simulink model "pure_pursuit_sl"  (R2019a)
settings: Solver=FixedStepDiscrete  StartTime=0.0  StopTime=inf  FixedStep=0.01  RelTol=1e-3
model workspace (MAT data in the model file):
  SL_ROS_VariableLengthArrays_MaxSizes.CommonInfo.ArrayTruncateAction = 'EmitWarning'
  SL_ROS_VariableLengthArrays_MaxSizes.MsgTypeMap = containers.Map
  SL_ROS_VariableLengthArrays_MaxSizes.MsgTypeMap.serialization.keys = {'autoware_msgs/Lane', 'autoware_msgs/lane', 'visualization_msgs/Marker'}
  SL_ROS_VariableLengthArrays_MaxSizes.MsgTypeMap.serialization.values{1}.PropertyName = 'Waypoints'
  SL_ROS_VariableLengthArrays_MaxSizes.MsgTypeMap.serialization.values{1}.DataType = 'autoware_msgs/Waypoint'
  SL_ROS_VariableLengthArrays_MaxSizes.MsgTypeMap.serialization.values{1}.MaxLength = 101
  SL_ROS_VariableLengthArrays_MaxSizes.MsgTypeMap.serialization.values{2}.PropertyName = 'Waypoints'
  SL_ROS_VariableLengthArrays_MaxSizes.MsgTypeMap.serialization.values{2}.DataType = 'autoware_msgs/waypoint'
  SL_ROS_VariableLengthArrays_MaxSizes.MsgTypeMap.serialization.values{2}.MaxLength = 101
  SL_ROS_VariableLengthArrays_MaxSizes.MsgTypeMap.serialization.values{3}(1).PropertyName = 'Colors'
  SL_ROS_VariableLengthArrays_MaxSizes.MsgTypeMap.serialization.values{3}(1).DataType = 'std_msgs/ColorRGBA'
  SL_ROS_VariableLengthArrays_MaxSizes.MsgTypeMap.serialization.values{3}(1).MaxLength = 80
  SL_ROS_VariableLengthArrays_MaxSizes.MsgTypeMap.serialization.values{3}(2).PropertyName = 'MeshResource'
  SL_ROS_VariableLengthArrays_MaxSizes.MsgTypeMap.serialization.values{3}(2).DataType = 'uint8'
  SL_ROS_VariableLengthArrays_MaxSizes.MsgTypeMap.serialization.values{3}(2).MaxLength = 128
  SL_ROS_VariableLengthArrays_MaxSizes.MsgTypeMap.serialization.values{3}(3).PropertyName = 'Ns'
  SL_ROS_VariableLengthArrays_MaxSizes.MsgTypeMap.serialization.values{3}(3).DataType = 'uint8'
  SL_ROS_VariableLengthArrays_MaxSizes.MsgTypeMap.serialization.values{3}(3).MaxLength = 128
  SL_ROS_VariableLengthArrays_MaxSizes.MsgTypeMap.serialization.values{3}(4).PropertyName = 'Points'
  SL_ROS_VariableLengthArrays_MaxSizes.MsgTypeMap.serialization.values{3}(4).DataType = 'geometry_msgs/Point'
  SL_ROS_VariableLengthArrays_MaxSizes.MsgTypeMap.serialization.values{3}(4).MaxLength = 80
  SL_ROS_VariableLengthArrays_MaxSizes.MsgTypeMap.serialization.values{3}(5).PropertyName = 'Text'
  SL_ROS_VariableLengthArrays_MaxSizes.MsgTypeMap.serialization.values{3}(5).DataType = 'uint8'
  SL_ROS_VariableLengthArrays_MaxSizes.MsgTypeMap.serialization.values{3}(5).MaxLength = 128
  SL_ROS_VariableLengthArrays_MaxSizes.MsgTypeMap.serialization.uniformity = 0
  SL_ROS_VariableLengthArrays_MaxSizes.MsgTypeMap.serialization.keyType = 'char'
  SL_ROS_VariableLengthArrays_MaxSizes.MsgTypeMap.serialization.valueType = 'any'
  is_pose_set_ = Simulink.Signal
  is_pose_set_.DataType = 'boolean'
  is_pose_set_.Dimensions = 1
  is_pose_set_.DimensionsMode = 'Fixed'
  is_pose_set_.Complexity = 'real'
  is_pose_set_.SampleTime = -1
  is_pose_set_.SamplingMode = 'auto'
  is_pose_set_.InitialValue = 'false'
  is_velocity_set_ = Simulink.Signal
  is_velocity_set_.DataType = 'boolean'
  is_velocity_set_.Dimensions = 1
  is_velocity_set_.DimensionsMode = 'Fixed'
  is_velocity_set_.Complexity = 'real'
  is_velocity_set_.SampleTime = -1
  is_velocity_set_.SamplingMode = 'auto'
  is_velocity_set_.InitialValue = 'false'
  is_waypoint_set_ = Simulink.Signal
  is_waypoint_set_.DataType = 'boolean'
  is_waypoint_set_.Dimensions = 1
  is_waypoint_set_.DimensionsMode = 'Fixed'
  is_waypoint_set_.Complexity = 'real'
  is_waypoint_set_.SampleTime = -1
  is_waypoint_set_.SamplingMode = 'auto'
  is_waypoint_set_.InitialValue = 'false'
  minimum_lookahead_distance = Simulink.Parameter
  minimum_lookahead_distance.Value = 6
  minimum_lookahead_distance.DataType = 'auto'
  minimum_lookahead_distance.Dimensions = [1 1]
undefined symbols (not defined in the file): Action, Color, Colors, Colors_SL_Info, FrameLocked, Header, Id, Ns, Points, Points_SL_Info, Pose, Scale, Twist, Type, X, Y, Z
libraries: robotlib x22, robotcorelib x4, simulink x1
(part 1 of 2)
settings Model: Creator=handai  LastModifiedBy=root
settings DataIOCC: SaveOutput=off  SignalLogging=off  DSMLogging=off  SaveTime=off  ReturnWorkspaceOutputs=off
settings DebuggingCC: PregeneratedLibrarySubsystemCodeDiagnostic=none  ArithmeticOperatorsInVariantConditions=warning
settings SFSimCC: SimUseLocalCustomCode=off
settings RTWCC: RTWUseLocalCustomCode=off

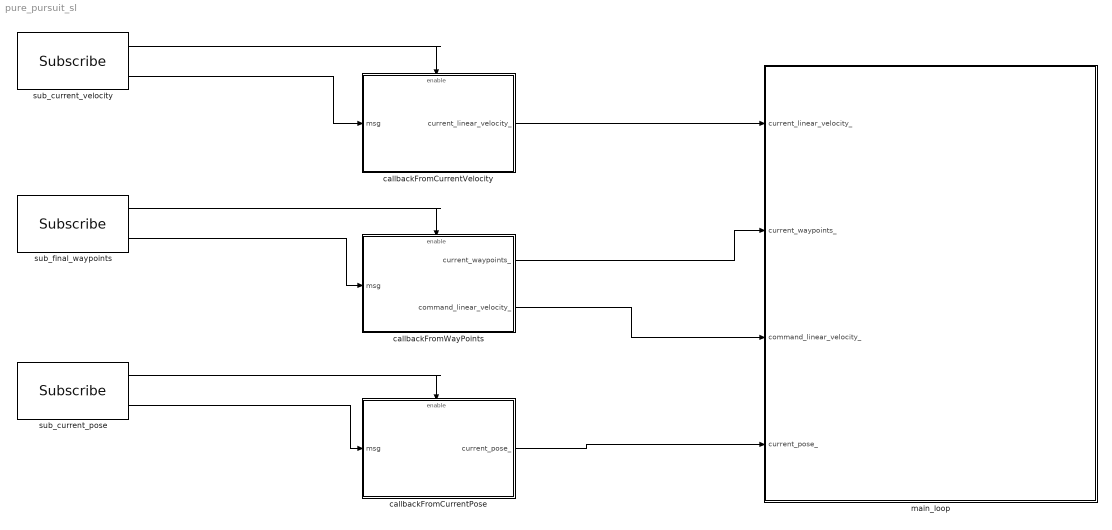
== system pure_pursuit_sl ==
  callbackFromCurrentPose : Subsystem
  callbackFromCurrentVelocity : Subsystem
  callbackFromWayPoints : Subsystem
  main_loop : Subsystem  TreatAsAtomicUnit=on  SystemSampleTime=0.03
      settings: AttributesFormatString=Ts = %<SystemSampleTime>[s]
  sub_current_pose : robotlib/Subscribe  topicSource=Specify your own  topic=/current_pose  messageType=geometry_msgs/PoseStamped  sampleTime=0.01  messageQueueLength=1
      settings: AttributesFormatString=Ts = %<sampleTime>[s]  SourceProductBaseCode=RO
  sub_current_velocity : robotlib/Subscribe  topicSource=Specify your own  topic=/current_velocity  messageType=geometry_msgs/TwistStamped  sampleTime=0.01  messageQueueLength=1
      settings: AttributesFormatString=Ts = %<sampleTime>[s]  SourceProductBaseCode=RO
  sub_final_waypoints : robotlib/Subscribe  topicSource=Specify your own  topic=/final_waypoints  messageType=autoware_msgs/Lane  sampleTime=-1  messageQueueLength=1
      settings: AttributesFormatString=Ts = %<sampleTime>[s]  SourceProductBaseCode=RO
  wires:
  sub_final_waypoints/1 -> callbackFromWayPoints/Enable
  sub_current_pose/2 -> callbackFromCurrentPose/1(msg)
  sub_current_pose/1 -> callbackFromCurrentPose/Enable
  sub_final_waypoints/2 -> callbackFromWayPoints/1(msg)
  callbackFromWayPoints/2(command_linear_velocity_) -> main_loop/3(command_linear_velocity_)
  sub_current_velocity/2 -> callbackFromCurrentVelocity/1(msg)
  sub_current_velocity/1 -> callbackFromCurrentVelocity/Enable
  callbackFromCurrentVelocity/1(current_linear_velocity_) -> main_loop/1(current_linear_velocity_)
  callbackFromWayPoints/1(current_waypoints_) -> main_loop/2(current_waypoints_)
  callbackFromCurrentPose/1(current_pose_) -> main_loop/4(current_pose_)

== system pure_pursuit_sl/callbackFromCurrentPose ==
  msg : Inport
  Enable : EnablePort
  Bus Selector : BusSelector  OutputSignals=Pose
  Constant : Constant  Value=true
  Data Store Write : DataStoreWrite  DataStoreName=is_pose_set_
  Signal Conversion1 : SignalConversion  OverrideOpt=off
  current_pose_ : Outport
  wires:
  Bus Selector/1 -> Signal Conversion1/1  "<Pose>"
  msg/1 -> Bus Selector/1
  Signal Conversion1/1 -> current_pose_/1  "current_pose_"
  Constant/1 -> Data Store Write/1

== system pure_pursuit_sl/callbackFromCurrentVelocity ==
  msg : Inport
  Enable : EnablePort
  Bus Selector1 : BusSelector  OutputSignals=Twist.Linear.X
  Constant : Constant  Value=true
  Data Store Write : DataStoreWrite  DataStoreName=is_velocity_set_
  Signal Conversion : SignalConversion  OverrideOpt=off
  current_linear_velocity_ : Outport
  wires:
  Bus Selector1/1 -> Signal Conversion/1  "<X>"
  msg/1 -> Bus Selector1/1
  Signal Conversion/1 -> current_linear_velocity_/1  "current_linear_velocity_"
  Constant/1 -> Data Store Write/1

== system pure_pursuit_sl/callbackFromWayPoints ==
  msg : Inport
  Enable : EnablePort
  Constant : Constant  Value=true
  Data Store Write : DataStoreWrite  DataStoreName=is_waypoint_set_
  Selector : Selector  IndexMode=Zero-based  InputPortWidth=101  IndexOptions=Index vector (port)  Indices=[1 3]  OutputSizes=1
  Signal Conversion2 : SignalConversion  OverrideOpt=off
  Signal Conversion3 : SignalConversion  OverrideOpt=off
  command_linear_velocity : BusSelector  OutputSignals=Twist.Twist.Linear.X
  idx : Constant  Value=0
  waypoint1 : BusSelector  OutputSignals=Waypoints
  current_waypoints_ : Outport
  command_linear_velocity_ : Outport  Port=2
  wires:
  waypoint1/1 -> Signal Conversion3/1, Selector/1  "<Waypoints>"
  Signal Conversion2/1 -> command_linear_velocity_/1  "command_linear_velocity_"
  idx/1 -> Selector/2
  command_linear_velocity/1 -> Signal Conversion2/1  "<X>"
  msg/1 -> waypoint1/1
  Selector/1 -> command_linear_velocity/1
  Signal Conversion3/1 -> current_waypoints_/1  "current_waypoints_"
  Constant/1 -> Data Store Write/1

== system pure_pursuit_sl/main_loop ==
  current_linear_velocity_ : Inport
  current_waypoints_ : Inport  Port=2
  command_linear_velocity_ : Inport  Port=3
  current_pose_ : Inport  Port=4
  Data Store Read : DataStoreRead  DataStoreName=is_pose_set_
  Data Store Read1 : DataStoreRead  DataStoreName=is_velocity_set_
  Data Store Read2 : DataStoreRead  DataStoreName=is_waypoint_set_
  If1 : If  NumInputs=3  IfExpression=u1 | u2 | u3
  Logical Operator : Logic  Operator=NOT  AllPortsSameDT=off  OutDataTypeStr=boolean
  Logical Operator1 : Logic  Operator=NOT  AllPortsSameDT=off  OutDataTypeStr=boolean
  Logical Operator2 : Logic  Operator=NOT  AllPortsSameDT=off  OutDataTypeStr=boolean
  loop_action : Subsystem  TreatAsAtomicUnit=on
  warn_messge : Subsystem  TreatAsAtomicUnit=on
  wires:
  Data Store Read/1 -> Logical Operator/1
  Data Store Read1/1 -> Logical Operator1/1
  Data Store Read2/1 -> Logical Operator2/1
  Logical Operator2/1 -> If1/3
  Logical Operator1/1 -> If1/2
  Logical Operator/1 -> If1/1
  If1/1 -> warn_messge/Action
  If1/2 -> loop_action/Action
  current_linear_velocity_/1 -> loop_action/1(current_linear_velocity_)
  current_waypoints_/1 -> loop_action/2(current_waypoints_)
  command_linear_velocity_/1 -> loop_action/3(command_linear_velocity_)
  current_pose_/1 -> loop_action/4(current_pose_)

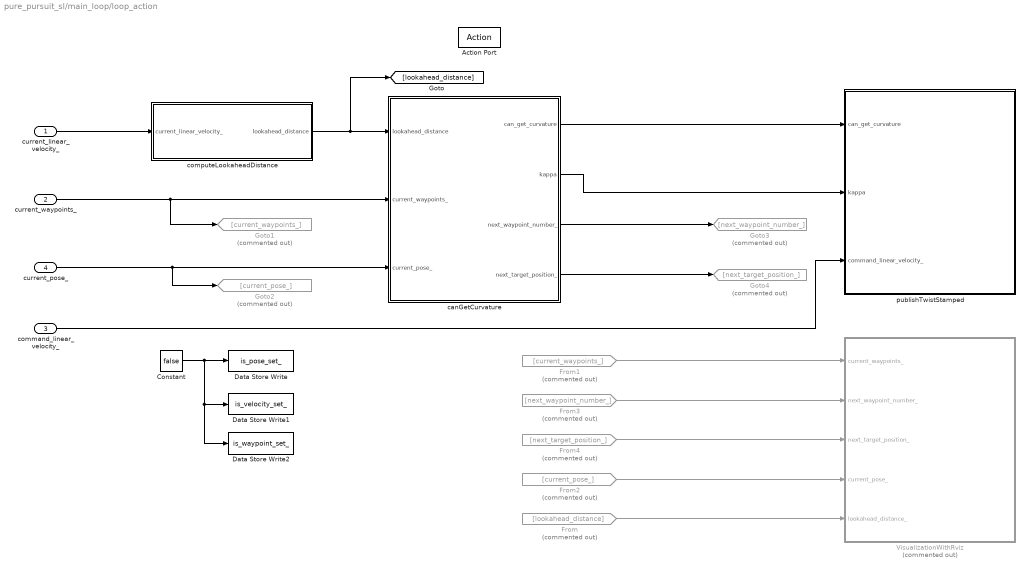
== system pure_pursuit_sl/main_loop/loop_action ==
  current_linear_velocity_ : Inport
  current_waypoints_ : Inport  Port=2
  command_linear_velocity_ : Inport  Port=3
  current_pose_ : Inport  Port=4
  Action Port : ActionPort  ActionPortLabel=else
  Constant : Constant  Priority=1000  Value=false
  Data Store Write : DataStoreWrite  DataStoreName=is_pose_set_
  Data Store Write1 : DataStoreWrite  DataStoreName=is_velocity_set_
  Data Store Write2 : DataStoreWrite  DataStoreName=is_waypoint_set_
  From : From  Commented=on  GotoTag=lookahead_distance
  From1 : From  Commented=on  GotoTag=current_waypoints_
  From2 : From  Commented=on  GotoTag=current_pose_
  From3 : From  Commented=on  GotoTag=next_waypoint_number_
  From4 : From  Commented=on  GotoTag=next_target_position_
  Goto1 : Goto  Commented=on  GotoTag=current_waypoints_
  Goto2 : Goto  Commented=on  GotoTag=current_pose_
  Goto3 : Goto  Commented=on  GotoTag=next_waypoint_number_
  Goto4 : Goto  Commented=on  GotoTag=next_target_position_
  VisualizationWithRviz : Subsystem  Priority=2000  Commented=on  TreatAsAtomicUnit=on
  canGetCurvature : Subsystem  TreatAsAtomicUnit=on
  computeLookaheadDistance : Subsystem  TreatAsAtomicUnit=on
  publishTwistStamped : Subsystem  Priority=1  TreatAsAtomicUnit=on
  wires:
  current_linear_velocity_/1 -> computeLookaheadDistance/1(current_linear_velocity_)
  computeLookaheadDistance/1(lookahead_distance) -> [lookahead_distance], canGetCurvature/1(lookahead_distance)
  current_waypoints_/1 -> Goto1/1, canGetCurvature/2(current_waypoints_)
  current_pose_/1 -> Goto2/1, canGetCurvature/3(current_pose_)
  canGetCurvature/1(can_get_curvature) -> publishTwistStamped/1(can_get_curvature)
  canGetCurvature/2(kappa) -> publishTwistStamped/2(kappa)
  command_linear_velocity_/1 -> publishTwistStamped/3(command_linear_velocity_)
  Constant/1 -> Data Store Write1/1, Data Store Write2/1, Data Store Write/1
  From/1 -> VisualizationWithRviz/5(lookahead_distance_)
  From1/1 -> VisualizationWithRviz/1(current_waypoints_)
  From2/1 -> VisualizationWithRviz/4(current_pose_)
  From3/1 -> VisualizationWithRviz/2(next_waypoint_number_)
  canGetCurvature/3(next_waypoint_number_) -> Goto3/1
  From4/1 -> VisualizationWithRviz/3(next_target_position_)
  canGetCurvature/4(next_target_position_) -> Goto4/1

== system pure_pursuit_sl/main_loop/warn_messge ==
  Action Port : ActionPort  ActionPortLabel=if(u1 | u2 | u3)
  MATLAB Function : MATLAB Function  TreatAsAtomicUnit=on

== system pure_pursuit_sl/main_loop/loop_action/VisualizationWithRviz ==
  note: advertise("trajectory_circle_mark")
  note: advertise("search_circle_mark")
  note: advertise("next_target_mark")
  note: advertise("next_waypoint_mark")
  current_waypoints_ : Inport
  next_waypoint_number_ : Inport  Port=2
  next_target_position_ : Inport  Port=3
  current_pose_ : Inport  Port=4
  lookahead_distance_ : Inport  Port=5
  Bus Selector : BusSelector  OutputSignals=Position
  Publish : robotlib/Publish  topicSource=Specify your own  topic=next_waypoint_mark  messageType=visualization_msgs/Marker  messageQueueLength=1
      settings: SourceProductBaseCode=RO
  Publish1 : robotlib/Publish  topicSource=Specify your own  topic=next_target_mark  messageType=visualization_msgs/Marker  messageQueueLength=1
      settings: SourceProductBaseCode=RO
  Publish2 : robotlib/Publish  topicSource=Specify your own  topic=search_circle_mark  messageType=visualization_msgs/Marker  messageQueueLength=1
      settings: SourceProductBaseCode=RO
  Publish3 : robotlib/Publish  topicSource=Specify your own  topic=trajectory_circle_mark  messageType=visualization_msgs/Marker  messageQueueLength=1
      settings: SourceProductBaseCode=RO
  displayNextTarget : Subsystem  TreatAsAtomicUnit=on
  displayNextWaypoint : Subsystem  TreatAsAtomicUnit=on
  displaySearchRadius : Subsystem  TreatAsAtomicUnit=on
  displayTrajectoryCircle : Subsystem  TreatAsAtomicUnit=on
  generateTrajectoryCircle : Subsystem  TreatAsAtomicUnit=on
  getPoseOfNextWaypoint : Subsystem  TreatAsAtomicUnit=on
  wires:
  current_waypoints_/1 -> getPoseOfNextWaypoint/1(current_waypoints_)
  next_waypoint_number_/1 -> getPoseOfNextWaypoint/2(next_waypoint_number_)
  getPoseOfNextWaypoint/1(pose_of_next_waypoint) -> displayNextWaypoint/1(pose_of_next_waypoint)
  displayNextWaypoint/1(marker) -> Publish/1
  next_target_position_/1 -> generateTrajectoryCircle/1(target), displayNextTarget/1(next_target_position_)
  displayNextTarget/1(marker) -> Publish1/1
  current_pose_/1 -> Bus Selector/1, generateTrajectoryCircle/2(current_pose_)
  Bus Selector/1 -> displaySearchRadius/1(current_pose)  "<Position>"
  lookahead_distance_/1 -> displaySearchRadius/2(search_radius)
  displaySearchRadius/1(marker) -> Publish2/1
  displayTrajectoryCircle/1(traj_circle) -> Publish3/1
  generateTrajectoryCircle/1(traj_circle_array) -> displayTrajectoryCircle/1(traj_circle_array)

== system pure_pursuit_sl/main_loop/loop_action/canGetCurvature ==
  lookahead_distance : Inport
  current_waypoints_ : Inport  Port=2
  current_pose_ : Inport  Port=3
  If : If  IfExpression=u1 == -1
  Merge : Merge
  curvature : Subsystem  TreatAsAtomicUnit=on
  getNextWaypoint : Subsystem  TreatAsAtomicUnit=on
  lost_next_waypoint : Subsystem  TreatAsAtomicUnit=on
  can_get_curvature : Outport
  kappa : Outport  Port=2
  next_waypoint_number_ : Outport  Port=3
  next_target_position_ : Outport  Port=4
  wires:
  curvature/1(can_get_curvature) -> Merge/2
  getNextWaypoint/1(next_waypoint_number_) -> next_waypoint_number_/1, curvature/1(nextWaypointNumber), If/1
  If/1 -> lost_next_waypoint/Action
  lookahead_distance/1 -> curvature/3(lookahead_distance), getNextWaypoint/1(lookahead_distance)
  curvature/2(kappa) -> kappa/1
  current_pose_/1 -> curvature/4(current_pose_Pose), getNextWaypoint/3(current_pose_Pose)
  lost_next_waypoint/1(can_get_curvaturet) -> Merge/1
  current_waypoints_/1 -> curvature/2(current_waypoints_), getNextWaypoint/2(current_waypoints_)
  If/2 -> curvature/Action
  Merge/1 -> can_get_curvature/1
  curvature/3(next_target_position_) -> next_target_position_/1

== system pure_pursuit_sl/main_loop/loop_action/computeLookaheadDistance ==
  current_linear_velocity_ : Inport
  If : If  NumInputs=3  IfExpression=u1 < u2  ElseIfExpressions=u1 > u3
  If Action Subsystem : Subsystem  TreatAsAtomicUnit=on
  If Action Subsystem1 : Subsystem  TreatAsAtomicUnit=on
  If Action Subsystem2 : Subsystem  TreatAsAtomicUnit=on
  Merge : Merge  Inputs=3
  lookadhead_distance_ratio : Gain  Gain=2.0
  maximum_lookahead_distance : Gain  Gain=10
  minimum_lookahead_distance : Constant  Value=minimum_lookahead_distance
  lookahead_distance : Outport
  wires:
  current_linear_velocity_/1 -> maximum_lookahead_distance/1, lookadhead_distance_ratio/1
  lookadhead_distance_ratio/1 -> If Action Subsystem2/1(In1), If/1  "ld"
  maximum_lookahead_distance/1 -> If Action Subsystem1/1(In1), If/3  "maximum_lookahead_distance"
  If Action Subsystem/1(Out1) -> Merge/1
  minimum_lookahead_distance/1 -> If Action Subsystem/1(In1), If/2
  Merge/1 -> lookahead_distance/1  "lookahead_distance"
  If Action Subsystem2/1(Out1) -> Merge/3
  If/1 -> If Action Subsystem/Action
  If Action Subsystem1/1(Out1) -> Merge/2
  If/3 -> If Action Subsystem2/Action
  If/2 -> If Action Subsystem1/Action

== system pure_pursuit_sl/main_loop/loop_action/publishTwistStamped ==
  can_get_curvature : Inport
  kappa : Inport  Port=2
  command_linear_velocity_ : Inport  Port=3
  Blank Message : robotlib/Blank Message  messageClass=Message  entityType=geometry_msgs/TwistStamped  messageType=geometry_msgs/TwistStamped  SampleTime=inf
      settings: SourceProductBaseCode=RO
  Bus Assignment : BusAssignment  AssignedSignals=Header.Stamp,Twist.Linear.X,Twist.Angular.Z
  Current Time : robotlib/Current Time  OutputFormat=bus  SampleTime=-1  ModelName=pure_pursuit_sl
      settings: SourceProductName=Robotics System Toolbox  SourceProductBaseCode=RO
  If Action Subsystem : Subsystem  TreatAsAtomicUnit=on
  If Action Subsystem1 : Subsystem  TreatAsAtomicUnit=on
  If1 : If  IfExpression=u1 == 1
  Merge1 : Merge
  Merge2 : Merge
  Publish : robotlib/Publish  topicSource=Specify your own  topic=/twist_raw  messageType=geometry_msgs/TwistStamped  messageQueueLength=1
      settings: SourceProductBaseCode=RO
  wires:
  Current Time/1 -> Bus Assignment/2
  Merge1/1 -> Bus Assignment/3
  Bus Assignment/1 -> Publish/1
  Merge2/1 -> Bus Assignment/4
  Blank Message/1 -> Bus Assignment/1
  If Action Subsystem1/1(linear) -> Merge1/2
  If1/1 -> If Action Subsystem/Action
  can_get_curvature/1 -> If1/1
  If Action Subsystem/1(linear) -> Merge1/1
  If Action Subsystem1/2(angular) -> Merge2/2
  kappa/1 -> If Action Subsystem/1(kappa)
  If1/2 -> If Action Subsystem1/Action
  If Action Subsystem/2(angular) -> Merge2/1
  command_linear_velocity_/1 -> If Action Subsystem/2(command_velocity)

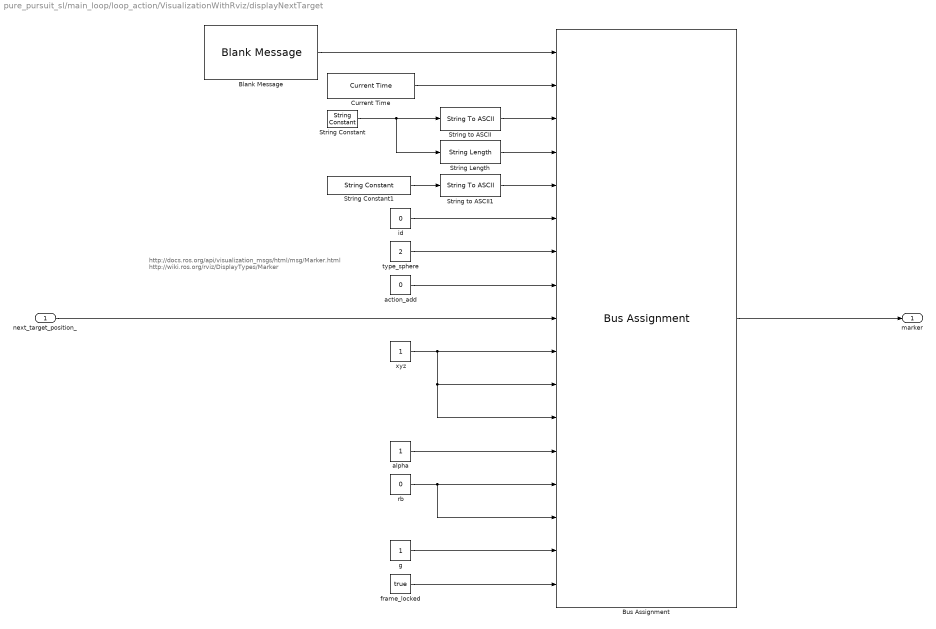
== system pure_pursuit_sl/main_loop/loop_action/VisualizationWithRviz/displayNextTarget ==
  note: http://docs.ros.org/api/visualization_msgs/html/msg/Marker.html
      | http://wiki.ros.org/rviz/DisplayTypes/Marker
  next_target_position_ : Inport
  Blank Message : robotlib/Blank Message  messageClass=Message  entityType=visualization_msgs/Marker  messageType=visualization_msgs/Marker  SampleTime=inf
      settings: SourceProductBaseCode=RO
  Bus Assignment : BusAssignment  AssignedSignals=Header.Stamp,Header.FrameId,Header.FrameId_SL_Info.CurrentLength,Ns,Id,Type,Action,Pose.Position,Scale.X,Scale.Y,Scale.Z,Color.A,Color.R,Color.B,Color.G,FrameLocked
  Current Time : robotlib/Current Time  OutputFormat=bus  SampleTime=-1  ModelName=pure_pursuit_sl
      settings: SourceProductName=Robotics System Toolbox  SourceProductBaseCode=RO
  String Constant : StringConstant  String="\"map\""
  String Constant1 : StringConstant  String="\"next_target_marker\""
  String Length : StringLength
  String to ASCII : StringToASCII  OutputVectorSize=128
  String to ASCII1 : StringToASCII  OutputVectorSize=128
  action_add : Constant  Value=0  OutDataTypeStr=int32
  alpha : Constant  OutDataTypeStr=single
  frame_locked : Constant  Value=true  OutDataTypeStr=boolean
  g : Constant  OutDataTypeStr=single
  id : Constant  Value=0  OutDataTypeStr=int32
  rb : Constant  Value=0  OutDataTypeStr=single
  type_sphere : Constant  Value=2  OutDataTypeStr=int32
  xyz : Constant  OutDataTypeStr=double
  marker : Outport
  wires:
  xyz/1 -> Bus Assignment/11, Bus Assignment/12, Bus Assignment/10
  String to ASCII/1 -> Bus Assignment/3
  type_sphere/1 -> Bus Assignment/7
  String Length/1 -> Bus Assignment/4
  String to ASCII1/1 -> Bus Assignment/5
  Blank Message/1 -> Bus Assignment/1
  String Constant1/1 -> String to ASCII1/1
  id/1 -> Bus Assignment/6
  frame_locked/1 -> Bus Assignment/17
  action_add/1 -> Bus Assignment/8
  alpha/1 -> Bus Assignment/13
  Bus Assignment/1 -> marker/1
  String Constant/1 -> String to ASCII/1, String Length/1
  rb/1 -> Bus Assignment/15, Bus Assignment/14
  Current Time/1 -> Bus Assignment/2
  next_target_position_/1 -> Bus Assignment/9
  g/1 -> Bus Assignment/16

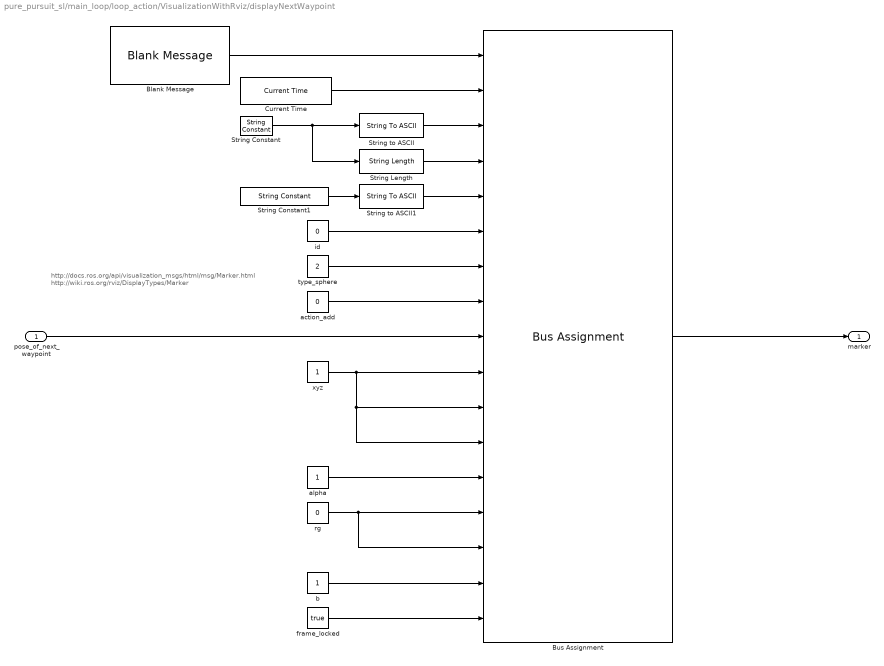
== system pure_pursuit_sl/main_loop/loop_action/VisualizationWithRviz/displayNextWaypoint ==
  note: http://docs.ros.org/api/visualization_msgs/html/msg/Marker.html
      | http://wiki.ros.org/rviz/DisplayTypes/Marker
  pose_of_next_waypoint : Inport
  Blank Message : robotlib/Blank Message  messageClass=Message  entityType=visualization_msgs/Marker  messageType=visualization_msgs/Marker  SampleTime=inf
      settings: SourceProductBaseCode=RO
  Bus Assignment : BusAssignment  AssignedSignals=Header.Stamp,Header.FrameId,Header.FrameId_SL_Info.CurrentLength,Ns,Id,Type,Action,Pose.Position,Scale.X,Scale.Y,Scale.Z,Color.A,Color.R,Color.G,Color.B,FrameLocked
  Current Time : robotlib/Current Time  OutputFormat=bus  SampleTime=-1  ModelName=pure_pursuit_sl
      settings: SourceProductName=Robotics System Toolbox  SourceProductBaseCode=RO
  String Constant : StringConstant  String='map'
  String Constant1 : StringConstant  String="\"next_waypoint_marker\""
  String Length : StringLength
  String to ASCII : StringToASCII  OutputVectorSize=128
  String to ASCII1 : StringToASCII  OutputVectorSize=128
  action_add : Constant  Value=0  OutDataTypeStr=int32
  alpha : Constant  OutDataTypeStr=single
  b : Constant  OutDataTypeStr=single
  frame_locked : Constant  Value=true  OutDataTypeStr=boolean
  id : Constant  Value=0  OutDataTypeStr=int32
  rg : Constant  Value=0  OutDataTypeStr=single
  type_sphere : Constant  Value=2  OutDataTypeStr=int32
  xyz : Constant  OutDataTypeStr=double
  marker : Outport
  wires:
  Blank Message/1 -> Bus Assignment/1
  Bus Assignment/1 -> marker/1
  pose_of_next_waypoint/1 -> Bus Assignment/9
  String Constant/1 -> String to ASCII/1, String Length/1
  String Length/1 -> Bus Assignment/4
  String Constant1/1 -> String to ASCII1/1
  String to ASCII/1 -> Bus Assignment/3
  String to ASCII1/1 -> Bus Assignment/5
  Current Time/1 -> Bus Assignment/2
  id/1 -> Bus Assignment/6
  xyz/1 -> Bus Assignment/11, Bus Assignment/12, Bus Assignment/10
  rg/1 -> Bus Assignment/15, Bus Assignment/14
  b/1 -> Bus Assignment/16
  frame_locked/1 -> Bus Assignment/17
  alpha/1 -> Bus Assignment/13
  type_sphere/1 -> Bus Assignment/7
  action_add/1 -> Bus Assignment/8

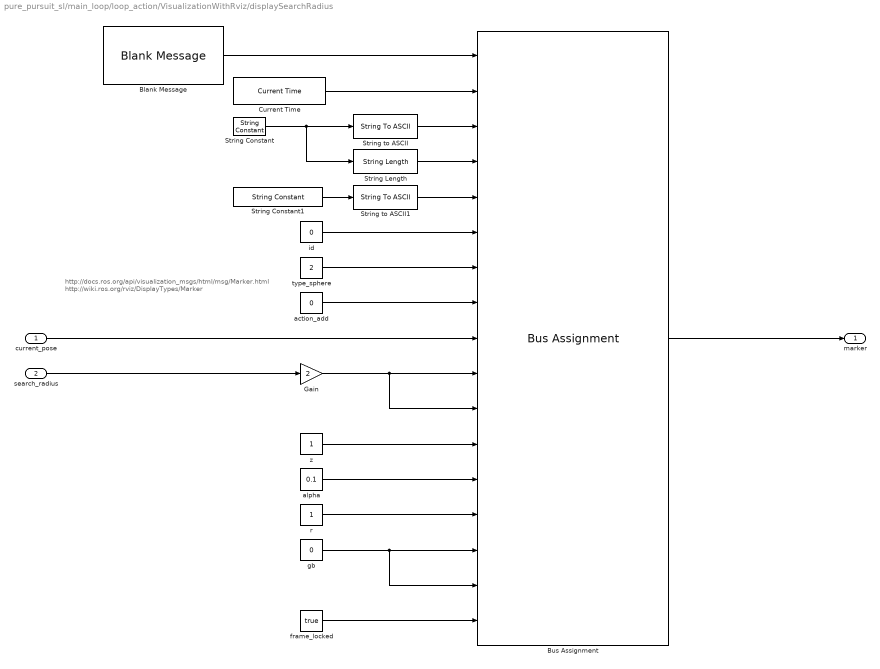
== system pure_pursuit_sl/main_loop/loop_action/VisualizationWithRviz/displaySearchRadius ==
  note: http://docs.ros.org/api/visualization_msgs/html/msg/Marker.html
      | http://wiki.ros.org/rviz/DisplayTypes/Marker
  current_pose : Inport
  search_radius : Inport  Port=2
  Blank Message : robotlib/Blank Message  messageClass=Message  entityType=visualization_msgs/Marker  messageType=visualization_msgs/Marker  SampleTime=inf
      settings: SourceProductBaseCode=RO
  Bus Assignment : BusAssignment  AssignedSignals=Header.Stamp,Header.FrameId,Header.FrameId_SL_Info.CurrentLength,Ns,Id,Type,Action,Pose.Position,Scale.X,Scale.Y,Scale.Z,Color.A,Color.R,Color.G,Color.B,FrameLocked
  Current Time : robotlib/Current Time  OutputFormat=bus  SampleTime=-1  ModelName=pure_pursuit_sl
      settings: SourceProductName=Robotics System Toolbox  SourceProductBaseCode=RO
  Gain : Gain  Gain=2
  String Constant : StringConstant  String="\"map\""
  String Constant1 : StringConstant  String="\"search_radius_marker\""
  String Length : StringLength
  String to ASCII : StringToASCII  OutputVectorSize=128
  String to ASCII1 : StringToASCII  OutputVectorSize=128
  action_add : Constant  Value=0  OutDataTypeStr=int32
  alpha : Constant  Value=0.1  OutDataTypeStr=single
  frame_locked : Constant  Value=true  OutDataTypeStr=boolean
  gb : Constant  Value=0  OutDataTypeStr=single
  id : Constant  Value=0  OutDataTypeStr=int32
  r : Constant  OutDataTypeStr=single
  type_sphere : Constant  Value=2  OutDataTypeStr=int32
  z : Constant  OutDataTypeStr=double
  marker : Outport
  wires:
  Current Time/1 -> Bus Assignment/2
  Bus Assignment/1 -> marker/1
  frame_locked/1 -> Bus Assignment/17
  alpha/1 -> Bus Assignment/13
  id/1 -> Bus Assignment/6
  String Constant1/1 -> String to ASCII1/1
  Blank Message/1 -> Bus Assignment/1
  String Length/1 -> Bus Assignment/4
  type_sphere/1 -> Bus Assignment/7
  z/1 -> Bus Assignment/12
  String Constant/1 -> String to ASCII/1, String Length/1
  gb/1 -> Bus Assignment/16, Bus Assignment/15
  String to ASCII/1 -> Bus Assignment/3
  action_add/1 -> Bus Assignment/8
  String to ASCII1/1 -> Bus Assignment/5
  current_pose/1 -> Bus Assignment/9
  search_radius/1 -> Gain/1
  Gain/1 -> Bus Assignment/11, Bus Assignment/10
  r/1 -> Bus Assignment/14

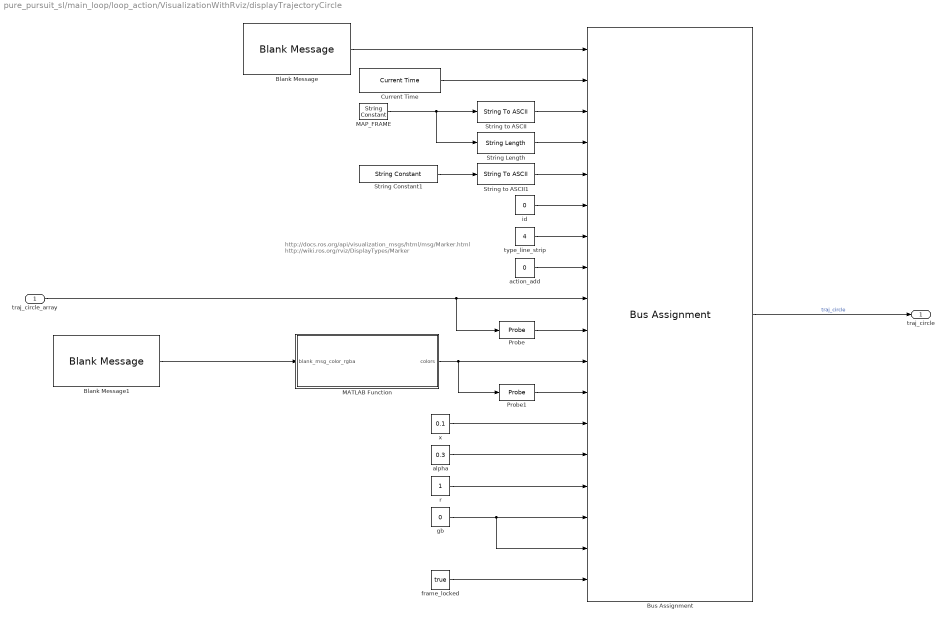
== system pure_pursuit_sl/main_loop/loop_action/VisualizationWithRviz/displayTrajectoryCircle ==
  note: http://docs.ros.org/api/visualization_msgs/html/msg/Marker.html
      | http://wiki.ros.org/rviz/DisplayTypes/Marker
  traj_circle_array : Inport
  Blank Message : robotlib/Blank Message  messageClass=Message  entityType=visualization_msgs/Marker  messageType=visualization_msgs/Marker  SampleTime=inf
      settings: SourceProductBaseCode=RO
  Blank Message1 : robotlib/Blank Message  messageClass=Message  entityType=std_msgs/ColorRGBA  messageType=std_msgs/ColorRGBA  SampleTime=inf
      settings: SourceProductBaseCode=RO
  Bus Assignment : BusAssignment  AssignedSignals=Header.Stamp,Header.FrameId,Header.FrameId_SL_Info.CurrentLength,Ns,Id,Type,Action,Points,Points_SL_Info.CurrentLength,Colors,Colors_SL_Info.CurrentLength,Scale.X,Color.A,Color.R,Color.G,Color.B,FrameLocked
  Current Time : robotlib/Current Time  OutputFormat=bus  SampleTime=-1  ModelName=pure_pursuit_sl
      settings: SourceProductName=Robotics System Toolbox  SourceProductBaseCode=RO
  MAP_FRAME : StringConstant  String="\"map\""
  MATLAB Function : MATLAB Function  TreatAsAtomicUnit=on
  Probe : Probe  ProbeWidth=off  ProbeSampleTime=off  ProbeComplexSignal=off  ProbeSignalDimensions=on  ProbeDimensionsDataType=uint32
  Probe1 : Probe  ProbeWidth=off  ProbeSampleTime=off  ProbeComplexSignal=off  ProbeSignalDimensions=on  ProbeDimensionsDataType=uint32
  String Constant1 : StringConstant  String="\"trajectory_circle_marker\""
  String Length : StringLength
  String to ASCII : StringToASCII  OutputVectorSize=128
  String to ASCII1 : StringToASCII  OutputVectorSize=128
  action_add : Constant  Value=0  OutDataTypeStr=int32
  alpha : Constant  Value=0.3  OutDataTypeStr=single
  frame_locked : Constant  Value=true  OutDataTypeStr=boolean
  gb : Constant  Value=0  OutDataTypeStr=single
  id : Constant  Value=0  OutDataTypeStr=int32
  r : Constant  OutDataTypeStr=single
  type_line_strip : Constant  Value=4  OutDataTypeStr=int32
  x : Constant  Value=0.1  OutDataTypeStr=double
  traj_circle : Outport
  wires:
  Current Time/1 -> Bus Assignment/2
  Bus Assignment/1 -> traj_circle/1  "traj_circle"
  id/1 -> Bus Assignment/6
  String Constant1/1 -> String to ASCII1/1
  Blank Message/1 -> Bus Assignment/1
  String Length/1 -> Bus Assignment/4
  type_line_strip/1 -> Bus Assignment/7
  MAP_FRAME/1 -> String to ASCII/1, String Length/1
  String to ASCII/1 -> Bus Assignment/3
  action_add/1 -> Bus Assignment/8
  String to ASCII1/1 -> Bus Assignment/5
  frame_locked/1 -> Bus Assignment/18
  x/1 -> Bus Assignment/13
  alpha/1 -> Bus Assignment/14
  r/1 -> Bus Assignment/15
  gb/1 -> Bus Assignment/17, Bus Assignment/16
  traj_circle_array/1 -> Bus Assignment/9, Probe/1
  Probe/1 -> Bus Assignment/10
  MATLAB Function/1(colors) -> Bus Assignment/11, Probe1/1
  Probe1/1 -> Bus Assignment/12
  Blank Message1/1 -> MATLAB Function/1(blank_msg_color_rgba)

== system pure_pursuit_sl/main_loop/loop_action/VisualizationWithRviz/generateTrajectoryCircle ==
  target : Inport
  current_pose_ : Inport  Port=2
  Blank Message : robotlib/Blank Message  messageClass=Message  entityType=geometry_msgs/Point  messageType=geometry_msgs/Point  SampleTime=inf
      settings: SourceProductBaseCode=RO
  MATLAB Function : MATLAB Function  TreatAsAtomicUnit=on
  calcRadius : Subsystem  TreatAsAtomicUnit=on
  traj_circle_array : Outport
  wires:
  target/1 -> calcRadius/1(target)
  current_pose_/1 -> MATLAB Function/3(current_pose), calcRadius/2(current_pose)
  calcRadius/1(radius) -> MATLAB Function/2(radius)
  Blank Message/1 -> MATLAB Function/1(blank_msg)
  MATLAB Function/1(traj_circle_array) -> traj_circle_array/1

== system pure_pursuit_sl/main_loop/loop_action/VisualizationWithRviz/getPoseOfNextWaypoint ==
  current_waypoints_ : Inport
  next_waypoint_number_ : Inport  Port=2
  Bus Selector : BusSelector  OutputSignals=Pose.Pose.Position
  Selector : Selector  IndexOptions=Index vector (port)  Indices=[1 3]  OutputSizes=1
  pose_of_next_waypoint : Outport
  wires:
  current_waypoints_/1 -> Selector/1
  Selector/1 -> Bus Selector/1
  next_waypoint_number_/1 -> Selector/2
  Bus Selector/1 -> pose_of_next_waypoint/1  "<Position>"

== system pure_pursuit_sl/main_loop/loop_action/canGetCurvature/curvature ==
  note: is_valid_curve is false
  note: is_valid_curve is true
  nextWaypointNumber : Inport  OutDataTypeStr=int32
  current_waypoints_ : Inport  Port=2
  lookahead_distance : Inport  Port=3
  current_pose_Pose : Inport  Port=4
  Action Port : ActionPort  ActionPortLabel=else
  If : If  IfExpression=u1 == 0
  Merge : Merge
  check whether curvature is valid or not : MATLAB Function  TreatAsAtomicUnit=on
  if is_linear_interpolation_ is false or next waypoint is first or last : Subsystem  TreatAsAtomicUnit=on
  is_not_valid_curve : Subsystem  TreatAsAtomicUnit=on
  minimum_lookahead_distance : Constant  Value=minimum_lookahead_distance
  can_get_curvature : Outport
  kappa : Outport  Port=2
  next_target_position_ : Outport  Port=3
  wires:
  nextWaypointNumber/1 -> if is_linear_interpolation_ is false or next waypoint is first or last/3(nextWaypointNumber)
  current_pose_Pose/1 -> check whether curvature is valid or not/1(current_pose_Pose), if is_linear_interpolation_ is false or next waypoint is first or last/2(current_pose_Pose)
  minimum_lookahead_distance/1 -> check whether curvature is valid or not/2(minimum_lookahead_distance)
  check whether curvature is valid or not/1(is_valid_curve) -> If/1
  If/1 -> is_not_valid_curve/Action
  If/2 -> if is_linear_interpolation_ is false or next waypoint is first or last/Action
  lookahead_distance/1 -> if is_linear_interpolation_ is false or next waypoint is first or last/4(lookahead_distance)
  is_not_valid_curve/1(return) -> Merge/1
  if is_linear_interpolation_ is false or next waypoint is first or last/1(return) -> Merge/2
  Merge/1 -> can_get_curvature/1
  if is_linear_interpolation_ is false or next waypoint is first or last/2(kappa) -> kappa/1
  current_waypoints_/1 -> if is_linear_interpolation_ is false or next waypoint is first or last/1(current_waypoint), check whether curvature is valid or not/3(waypoint)
  if is_linear_interpolation_ is false or next waypoint is first or last/3(next_target_position_) -> next_target_position_/1

== system pure_pursuit_sl/main_loop/loop_action/canGetCurvature/getNextWaypoint ==
  note: 1ベースの信号
  lookahead_distance : Inport
  current_waypoints_ : Inport  Port=2
  current_pose_Pose : Inport  Port=3
  If : If  IfExpression=u1 == 0
  If Action Subsystem : Subsystem  TreatAsAtomicUnit=on
  If Action Subsystem1 : Subsystem  TreatAsAtomicUnit=on
  Merge : Merge
  path_size : Probe  ProbeSampleTime=off  ProbeComplexSignal=off  ProbeWidthDataType=int32
  next_waypoint_number_ : Outport
  wires:
  current_waypoints_/1 -> If Action Subsystem1/2(current_waypoint), path_size/1
  If Action Subsystem/1(return) -> Merge/1
  If/1 -> If Action Subsystem/Action
  lookahead_distance/1 -> If Action Subsystem1/4(Iookahead_distance)
  current_pose_Pose/1 -> If Action Subsystem1/3(current_pose_Pose)
  If Action Subsystem1/1(return) -> Merge/2
  If/2 -> If Action Subsystem1/Action
  Merge/1 -> next_waypoint_number_/1  "next_waypoint_number_"
  path_size/1 -> If Action Subsystem1/1(path_size), If/1  "path_size"

== system pure_pursuit_sl/main_loop/loop_action/canGetCurvature/lost_next_waypoint ==
  Action Port : ActionPort  ActionPortLabel=if(u1 == -1)
  Constant : Constant  Value=false  OutDataTypeStr=boolean
  MATLAB Function : MATLAB Function  TreatAsAtomicUnit=on
  can_get_curvaturet : Outport  InitialOutput=false
  wires:
  Constant/1 -> can_get_curvaturet/1

== system pure_pursuit_sl/main_loop/loop_action/computeLookaheadDistance/If Action Subsystem ==
  In1 : Inport
  Action Port : ActionPort  ActionPortLabel=if(u1 < u2)
  Out1 : Outport
  wires:
  In1/1 -> Out1/1

== system pure_pursuit_sl/main_loop/loop_action/computeLookaheadDistance/If Action Subsystem1 ==
  In1 : Inport
  Action Port : ActionPort  ActionPortLabel=elseif(u1 > u3)
  Out1 : Outport
  wires:
  In1/1 -> Out1/1

== system pure_pursuit_sl/main_loop/loop_action/computeLookaheadDistance/If Action Subsystem2 ==
  In1 : Inport
  Action Port : ActionPort  ActionPortLabel=else
  Out1 : Outport
  wires:
  In1/1 -> Out1/1

== system pure_pursuit_sl/main_loop/loop_action/publishTwistStamped/If Action Subsystem ==
  kappa : Inport
  command_velocity : Inport  Port=2
  Action Port : ActionPort  ActionPortLabel=if(u1 == 1)
  Product : Product
  linear : Outport
  angular : Outport  Port=2
  wires:
  command_velocity/1 -> Product/1, linear/1
  kappa/1 -> Product/2
  Product/1 -> angular/1

== system pure_pursuit_sl/main_loop/loop_action/publishTwistStamped/If Action Subsystem1 ==
  Action Port : ActionPort  ActionPortLabel=else
  Constant : Constant  Value=0
  Constant1 : Constant  Value=0
  linear : Outport
  angular : Outport  Port=2
  wires:
  Constant/1 -> linear/1
  Constant1/1 -> angular/1

== system pure_pursuit_sl/main_loop/loop_action/VisualizationWithRviz/generateTrajectoryCircle/calcRadius ==
  target : Inport
  current_pose : Inport  Port=2
  Bus Selector : BusSelector  OutputSignals=Position
  Gain : Gain  Gain=2
  If : If  IfExpression=u1 ~= 0
  Merge : Merge
  calcRadius : Subsystem  TreatAsAtomicUnit=on
  calcRelativeCoordinate : Subsystem  TreatAsAtomicUnit=on
  getPlaneDistance : Subsystem  TreatAsAtomicUnit=on
  numerator : Math  Operator=square  SaturateOnIntegerOverflow=on
  point_y : Selector  InputPortWidth=4  IndexOptions=Index vector (port)  Indices=[1 3]  OutputSizes=1
  radius_zero : Subsystem  TreatAsAtomicUnit=on
  select_y : Constant  Value=2
  radius : Outport
  wires:
  target/1 -> getPlaneDistance/2(target1), calcRelativeCoordinate/1(target)
  current_pose/1 -> Bus Selector/1, calcRelativeCoordinate/2(current_pose_)
  select_y/1 -> point_y/2
  point_y/1 -> Gain/1
  calcRelativeCoordinate/1(tf_point_msg) -> point_y/1
  Gain/1 -> calcRadius/2(denominator), If/1  "denominator"
  getPlaneDistance/1(Distance) -> numerator/1
  Bus Selector/1 -> getPlaneDistance/1(target2)  "<Position>"
  numerator/1 -> calcRadius/1(numerator)  "numerator"
  If/1 -> calcRadius/Action
  If/2 -> radius_zero/Action
  Merge/1 -> radius/1
  calcRadius/1(radius) -> Merge/1
  radius_zero/1(radius) -> Merge/2

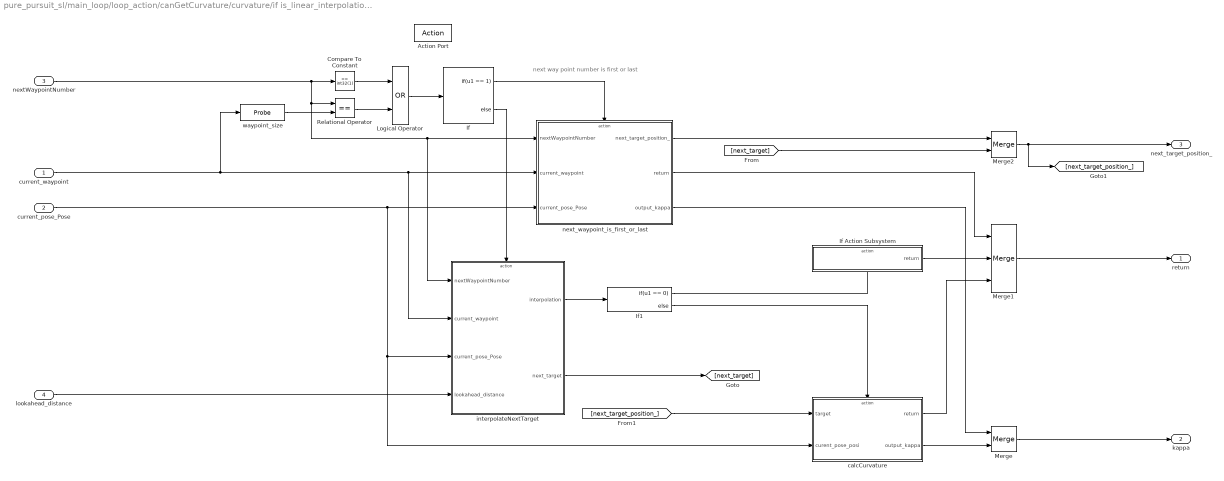
== system pure_pursuit_sl/main_loop/loop_action/canGetCurvature/curvature/if is_linear_interpolation_ is false or next waypoint is first or last ==
  note: next way point number is first or last
  current_waypoint : Inport
  current_pose_Pose : Inport  Port=2
  nextWaypointNumber : Inport  Port=3
  lookahead_distance : Inport  Port=4
  Action Port : ActionPort  ActionPortLabel=else
  " next_waypoint_is_first_or_last" : Subsystem  TreatAsAtomicUnit=on
  Compare To Constant : simulink/Logic and Bit Operations/Compare To Constant  relop===  const=int32(1)  OutDataTypeStr=boolean
  If : If  IfExpression=u1 == 1
  If Action Subsystem : Subsystem  TreatAsAtomicUnit=on
  If1 : If  IfExpression=u1 == 0
  Logical Operator : Logic  Operator=OR  AllPortsSameDT=off  OutDataTypeStr=boolean
  Merge : Merge
  Merge1 : Merge  Inputs=3
  Merge2 : Merge
  Relational Operator : RelationalOperator  Operator===  OutDataTypeStr=boolean  RndMeth=Simplest
  calcCurvature : Subsystem  TreatAsAtomicUnit=on
  interpolateNextTarget : Subsystem  Description=|  TreatAsAtomicUnit=on
      | linear interpolation and
      | calculate angular velocity
      settings: AttributesFormatString=%<Description>
  waypoint_size : Probe  ProbeSampleTime=off  ProbeComplexSignal=off  ProbeWidthDataType=int32
  return : Outport
  kappa : Outport  Port=2
  next_target_position_ : Outport  Port=3
  wires:
  nextWaypointNumber/1 -> Compare To Constant/1, interpolateNextTarget/1(nextWaypointNumber), " next_waypoint_is_first_or_last"/1(nextWaypointNumber), Relational Operator/1
  If/1 -> " next_waypoint_is_first_or_last"/Action
  current_waypoint/1 -> waypoint_size/1, interpolateNextTarget/2(current_waypoint), " next_waypoint_is_first_or_last"/2(current_waypoint)
  current_pose_Pose/1 -> interpolateNextTarget/3(current_pose_Pose), calcCurvature/2(curent_pose_posi), " next_waypoint_is_first_or_last"/3(current_pose_Pose)
  lookahead_distance/1 -> interpolateNextTarget/4(lookahead_distance)
  If/2 -> interpolateNextTarget/Action
  Merge/1 -> kappa/1
  " next_waypoint_is_first_or_last"/3(output_kappa) -> Merge/1
  " next_waypoint_is_first_or_last"/2(return) -> Merge1/1
  Merge1/1 -> return/1
  waypoint_size/1 -> Relational Operator/2
  Compare To Constant/1 -> Logical Operator/1
  Relational Operator/1 -> Logical Operator/2
  Logical Operator/1 -> If/1
  interpolateNextTarget/1(interpolation) -> If1/1
  If Action Subsystem/1(return) -> Merge1/2
  If1/1 -> If Action Subsystem/Action
  If1/2 -> calcCurvature/Action
  calcCurvature/2(output_kappa) -> Merge/2
  calcCurvature/1(return) -> Merge1/3
  " next_waypoint_is_first_or_last"/1(next_target_position_) -> Merge2/1
  [next_target] -> Merge2/2
  Merge2/1 -> [next_target_position_], next_target_position_/1
  interpolateNextTarget/2(next_target) -> [next_target]
  [next_target_position_] -> calcCurvature/1(target)

== system pure_pursuit_sl/main_loop/loop_action/canGetCurvature/curvature/is_not_valid_curve ==
  Action Port : ActionPort  ActionPortLabel=if(u1 == 0)
  Constant : Constant  Value=false  OutDataTypeStr=boolean
  return : Outport
  wires:
  Constant/1 -> return/1

== system pure_pursuit_sl/main_loop/loop_action/canGetCurvature/getNextWaypoint/If Action Subsystem ==
  Action Port : ActionPort  ActionPortLabel=if(u1 == 0)
  next_waypoint_number_ : Constant  Value=-1  OutDataTypeStr=int32
  return : Outport  InitialOutput=-1
  wires:
  next_waypoint_number_/1 -> return/1  "next_waypoint_number_"

== system pure_pursuit_sl/main_loop/loop_action/canGetCurvature/getNextWaypoint/If Action Subsystem1 ==
  path_size : Inport
  current_waypoint : Inport  Port=2
  current_pose_Pose : Inport  Port=3
  Iookahead_distance : Inport  Port=4
  Action Port : ActionPort  ActionPortLabel=else
  MATLAB Function : MATLAB Function  TreatAsAtomicUnit=on
  return : Outport
  wires:
  current_waypoint/1 -> MATLAB Function/4(waypoint)
  current_pose_Pose/1 -> MATLAB Function/2(current_pose_Pose)
  Iookahead_distance/1 -> MATLAB Function/3(lookahead_distance)
  path_size/1 -> MATLAB Function/1(path_size)
  MATLAB Function/1(next_waypoint_number) -> return/1

== system pure_pursuit_sl/main_loop/loop_action/VisualizationWithRviz/generateTrajectoryCircle/calcRadius/calcRadius ==
  numerator : Inport
  denominator : Inport  Port=2
  Action Port : ActionPort  ActionPortLabel=if(u1 ~= 0)
  Divide : Product  Inputs=*/
  radius : Outport
  wires:
  numerator/1 -> Divide/1
  denominator/1 -> Divide/2
  Divide/1 -> radius/1

== system pure_pursuit_sl/main_loop/loop_action/VisualizationWithRviz/generateTrajectoryCircle/calcRadius/calcRelativeCoordinate ==
  target : Inport
  current_pose_ : Inport  Port=2
  Bus Selector : BusSelector  OutputSignals=Orientation.W,Orientation.X,Orientation.Y,Orientation.Z
  Bus Selector1 : BusSelector  OutputSignals=Position.X,Position.Y,Position.Z
  Bus Selector3 : BusSelector  OutputSignals=X,Y,Z
  Constant : Constant
  Coordinate Transformation Conversion : robotcorelib/Coordinate Transformation Conversion  InputRepresentation=Quaternion  InputEulerSequence=XYZ  ShowTrVecInputPort=on  OutputRepresentation=Homogeneous Transformation  OutputEulerSequence=ZYX  ShowTrVecOutputPort=on  SimulateUsing=Interpreted execution
      settings: SourceProductBaseCode=RO
  Position Vector : Concatenate  NumInputs=3
  Product : Product  Inputs=/  Multiplication=Matrix(*)
  Product1 : Product  Multiplication=Matrix(*)
  "Quaternion Vector " : Concatenate  NumInputs=4
  point : Concatenate  NumInputs=4
  tf_point_msg : Outport
  wires:
  current_pose_/1 -> Bus Selector/1, Bus Selector1/1
  Position Vector/1 -> Coordinate Transformation Conversion/2
  Bus Selector1/3 -> Position Vector/3  "<Z>"
  "Quaternion Vector "/1 -> Coordinate Transformation Conversion/1
  Bus Selector1/2 -> Position Vector/2  "<Y>"
  Bus Selector1/1 -> Position Vector/1  "<X>"
  Coordinate Transformation Conversion/1 -> Product/1
  Product/1 -> Product1/1
  target/1 -> Bus Selector3/1
  Bus Selector3/2 -> point/2  "<Y>"
  Bus Selector3/3 -> point/3  "<Z>"
  Bus Selector3/1 -> point/1  "<X>"
  point/1 -> Product1/2
  Product1/1 -> tf_point_msg/1  "tf_point_msg"
  Bus Selector/1 -> "Quaternion Vector "/1  "<W>"
  Bus Selector/2 -> "Quaternion Vector "/2  "<X>"
  Bus Selector/3 -> "Quaternion Vector "/3  "<Y>"
  Bus Selector/4 -> "Quaternion Vector "/4  "<Z>"
  Constant/1 -> point/4

== system pure_pursuit_sl/main_loop/loop_action/VisualizationWithRviz/generateTrajectoryCircle/calcRadius/getPlaneDistance ==
  target2 : Inport
  target1 : Inport  Port=2
  Add : Sum
  Bus Selector1 : BusSelector  OutputSignals=X,Y
  Bus Selector2 : BusSelector  OutputSignals=X,Y
  Math Function : Math  Operator=square  SaturateOnIntegerOverflow=on
  Math Function1 : Math  Operator=square  SaturateOnIntegerOverflow=on
  Sqrt : Sqrt  SaturateOnIntegerOverflow=on
  Subtract : Sum  Inputs=+-
  Subtract1 : Sum  Inputs=+-
  Distance : Outport
  wires:
  Subtract1/1 -> Math Function/1
  target2/1 -> Bus Selector1/1
  Bus Selector1/1 -> Subtract1/2  "<X>"
  target1/1 -> Bus Selector2/1
  Add/1 -> Sqrt/1
  Bus Selector2/1 -> Subtract1/1  "<X>"
  Bus Selector2/2 -> Subtract/1  "<Y>"
  Sqrt/1 -> Distance/1
  Math Function/1 -> Add/1
  Subtract/1 -> Math Function1/1
  Math Function1/1 -> Add/2
  Bus Selector1/2 -> Subtract/2  "<Y>"

== system pure_pursuit_sl/main_loop/loop_action/VisualizationWithRviz/generateTrajectoryCircle/calcRadius/radius_zero ==
  Action Port : ActionPort  ActionPortLabel=else
  Constant : Constant  Value=0
  radius : Outport
  wires:
  Constant/1 -> radius/1

== system pure_pursuit_sl/main_loop/loop_action/canGetCurvature/curvature/if is_linear_interpolation_ is false or next waypoint is first or last/ next_waypoint_is_first_or_last ==
  nextWaypointNumber : Inport
  current_waypoint : Inport  Port=2
  current_pose_Pose : Inport  Port=3
  Action Port : ActionPort  ActionPortLabel=if(u1 == 1)
  Bus Selector : BusSelector  OutputSignals=Pose.Pose.Position
  Constant1 : Constant  Value=true  OutDataTypeStr=boolean
  Signal Conversion : SignalConversion  OverrideOpt=off
  calcCurvature : Subsystem  TreatAsAtomicUnit=on
  next_target_position : Selector  InputPortWidth=101  IndexOptions=Index vector (port)  Indices=[1 3]  OutputSizes=1
  next_target_position_ : Outport
  return : Outport  Port=2  InitialOutput=true
  output_kappa : Outport  Port=3
  wires:
  current_waypoint/1 -> next_target_position/1
  nextWaypointNumber/1 -> next_target_position/2
  next_target_position/1 -> Bus Selector/1
  current_pose_Pose/1 -> calcCurvature/2(current_pose_Pose)
  Bus Selector/1 -> Signal Conversion/1  "<Position>"
  Constant1/1 -> return/1
  calcCurvature/1(output_kappa) -> output_kappa/1
  Signal Conversion/1 -> next_target_position_/1, calcCurvature/1(target)  "next_target_position_"

== system pure_pursuit_sl/main_loop/loop_action/canGetCurvature/curvature/if is_linear_interpolation_ is false or next waypoint is first or last/If Action Subsystem ==
  Action Port : ActionPort  ActionPortLabel=if(u1 == 0)
  Constant : Constant  Value=false
  MATLAB Function : MATLAB Function  TreatAsAtomicUnit=on
  return : Outport  InitialOutput=false
  wires:
  Constant/1 -> return/1

== system pure_pursuit_sl/main_loop/loop_action/canGetCurvature/curvature/if is_linear_interpolation_ is false or next waypoint is first or last/calcCurvature ==
  target : Inport
  curent_pose_posi : Inport  Port=2
  Action Port : ActionPort  ActionPortLabel=else
  Constant : Constant  Value=true
  calcCurvature : Subsystem  TreatAsAtomicUnit=on
  return : Outport
  output_kappa : Outport  Port=2
  wires:
  calcCurvature/1(output_kappa) -> output_kappa/1
  target/1 -> calcCurvature/1(target)
  curent_pose_posi/1 -> calcCurvature/2(current_pose_Pose)
  Constant/1 -> return/1

== system pure_pursuit_sl/main_loop/loop_action/canGetCurvature/curvature/if is_linear_interpolation_ is false or next waypoint is first or last/interpolateNextTarget ==
  nextWaypointNumber : Inport
  current_waypoint : Inport  Port=2
  current_pose_Pose : Inport  Port=3
  lookahead_distance : Inport  Port=4
  Action Port : ActionPort  ActionPortLabel=else
  If2 : If  IfExpression=u1
  Merge : Merge
  Merge1 : Merge
  NextWaypoint_equal_PathSize : Subsystem  TreatAsAtomicUnit=on
  Relational Operator : RelationalOperator  Operator===  OutDataTypeStr=boolean  RndMeth=Simplest
  Subsystem : Subsystem
  path_size : Probe  ProbeSampleTime=off  ProbeComplexSignal=off  ProbeWidthDataType=int32
  interpolation : Outport
  next_target : Outport  Port=2
  wires:
  current_waypoint/1 -> NextWaypoint_equal_PathSize/2(current_waypoint), Subsystem/2(current_waypoint), path_size/1
  nextWaypointNumber/1 -> Subsystem/1(nextWaypointNumber), Relational Operator/1, NextWaypoint_equal_PathSize/1(nextWaypointNumber)
  path_size/1 -> Relational Operator/2
  Relational Operator/1 -> If2/1
  If2/1 -> NextWaypoint_equal_PathSize/Action
  lookahead_distance/1 -> Subsystem/3(lookahead_distance)
  current_pose_Pose/1 -> Subsystem/4(current_pose_Pose)
  If2/2 -> Subsystem/Action
  NextWaypoint_equal_PathSize/1(next_target) -> Merge/1
  Subsystem/1(next_target) -> Merge/2
  Merge/1 -> next_target/1
  Merge1/1 -> interpolation/1
  Subsystem/2(return) -> Merge1/2
  NextWaypoint_equal_PathSize/2(return) -> Merge1/1

== system pure_pursuit_sl/main_loop/loop_action/canGetCurvature/curvature/if is_linear_interpolation_ is false or next waypoint is first or last/ next_waypoint_is_first_or_last/calcCurvature ==
  target : Inport
  current_pose_Pose : Inport  Port=2
  Constant : Constant
  Divide : Product  Inputs=*/
  Gain : Gain  Gain=2
  If : If  NumInputs=2  IfExpression=u1 ~= 0  ElseIfExpressions=u2 > 0
  Merge : Merge  Inputs=3
  RADIUS_MAX : Constant  Value=90000000000
  calcRelativeCoordinate : Subsystem  TreatAsAtomicUnit=on
  denominator : Math  Operator=square  SaturateOnIntegerOverflow=on
  getPlaneDistance : Subsystem  TreatAsAtomicUnit=on
  minus_KAPPA_MIN : Subsystem  TreatAsAtomicUnit=on
  num_div_den : Subsystem  TreatAsAtomicUnit=on
  plus_KAPPA_MIN : Subsystem  TreatAsAtomicUnit=on
  point_y : Selector  InputPortWidth=4  IndexOptions=Index vector (port)  Indices=[1 3]  OutputSizes=1
  select_y : Constant  Value=2
  output_kappa : Outport
  wires:
  calcRelativeCoordinate/1(ros_pose) -> point_y/1
  If/1 -> num_div_den/Action
  point_y/1 -> Gain/1
  num_div_den/1(kappa) -> Merge/1
  getPlaneDistance/1(Distance) -> denominator/1
  target/1 -> calcRelativeCoordinate/1(target), getPlaneDistance/1(target1)
  Merge/1 -> output_kappa/1
  current_pose_Pose/1 -> getPlaneDistance/2(target2), calcRelativeCoordinate/2(current_pose_)
  denominator/1 -> If/1, num_div_den/1(denominator)  "denominator"
  select_y/1 -> point_y/2
  Gain/1 -> If/2, num_div_den/2(numerator)  "numerator"
  If/3 -> minus_KAPPA_MIN/Action
  minus_KAPPA_MIN/1(Out1) -> Merge/3
  plus_KAPPA_MIN/1(Out1) -> Merge/2
  If/2 -> plus_KAPPA_MIN/Action
  RADIUS_MAX/1 -> Divide/2
  Divide/1 -> minus_KAPPA_MIN/1(In1), plus_KAPPA_MIN/1(In1)  "KAPPA_MIN_"
  Constant/1 -> Divide/1

== system pure_pursuit_sl/main_loop/loop_action/canGetCurvature/curvature/if is_linear_interpolation_ is false or next waypoint is first or last/calcCurvature/calcCurvature ==
  target : Inport
  current_pose_Pose : Inport  Port=2
  Constant : Constant
  Divide : Product  Inputs=*/
  Gain : Gain  Gain=2
  If : If  NumInputs=2  IfExpression=u1 ~= 0  ElseIfExpressions=u2 > 0
  Merge : Merge  Inputs=3
  RADIUS_MAX : Constant  Value=90000000000
  calcRelativeCoordinate : Subsystem  TreatAsAtomicUnit=on
  denominator : Math  Operator=square  SaturateOnIntegerOverflow=on
  getPlaneDistance : Subsystem  TreatAsAtomicUnit=on
  minus_KAPPA_MIN : Subsystem  TreatAsAtomicUnit=on
  num_div_den : Subsystem  TreatAsAtomicUnit=on
  plus_KAPPA_MIN : Subsystem  TreatAsAtomicUnit=on
  point_y : Selector  InputPortWidth=4  IndexOptions=Index vector (port)  Indices=[1 3]  OutputSizes=1
  select_y : Constant  Value=2
  output_kappa : Outport
  wires:
  calcRelativeCoordinate/1(ros_pose) -> point_y/1
  If/1 -> num_div_den/Action
  point_y/1 -> Gain/1
  num_div_den/1(kappa) -> Merge/1
  getPlaneDistance/1(Distance) -> denominator/1
  target/1 -> calcRelativeCoordinate/1(target), getPlaneDistance/1(target1)
  Merge/1 -> output_kappa/1
  current_pose_Pose/1 -> getPlaneDistance/2(target2), calcRelativeCoordinate/2(current_pose_)
  denominator/1 -> If/1, num_div_den/1(denominator)  "denominator"
  select_y/1 -> point_y/2
  Gain/1 -> If/2, num_div_den/2(numerator)  "numerator"
  If/3 -> minus_KAPPA_MIN/Action
  minus_KAPPA_MIN/1(Out1) -> Merge/3
  plus_KAPPA_MIN/1(Out1) -> Merge/2
  If/2 -> plus_KAPPA_MIN/Action
  RADIUS_MAX/1 -> Divide/2
  Divide/1 -> minus_KAPPA_MIN/1(In1), plus_KAPPA_MIN/1(In1)  "KAPPA_MIN_"
  Constant/1 -> Divide/1

== system pure_pursuit_sl/main_loop/loop_action/canGetCurvature/curvature/if is_linear_interpolation_ is false or next waypoint is first or last/interpolateNextTarget/NextWaypoint_equal_PathSize ==
  nextWaypointNumber : Inport
  current_waypoint : Inport  Port=2
  Action Port : ActionPort  ActionPortLabel=if(u1)
  Bus Selector : BusSelector  OutputSignals=Pose.Pose.Position
  Constant1 : Constant  Value=true  OutDataTypeStr=boolean
  end : Selector  InputPortWidth=101  IndexOptions=Index vector (port)  Indices=[1 3]  OutputSizes=1
  next_target : Outport
  return : Outport  Port=2  InitialOutput=true
  wires:
  Constant1/1 -> return/1
  current_waypoint/1 -> end/1
  nextWaypointNumber/1 -> end/2
  end/1 -> Bus Selector/1
  Bus Selector/1 -> next_target/1  "<Position>"
